simulink model "Foc_2024b"  (R2025a)
settings: Solver=FixedStepDiscrete  StartTime=0.0  StopTime=10.0  FixedStep=0.001  RelTol=1e-3
values from neighbouring files (symbols this model uses):
  cal_AdcMaxCountsHw = NoneSAR.Parameter    [Foc_2024b_LoadCalParameter.m]
  cal_AdcRefVoltHw = NoneSAR.Parameter    [Foc_2024b_LoadCalParameter.m]
  cal_AdcVoltMidHw = NoneSAR.Parameter    [Foc_2024b_LoadCalParameter.m]
  cal_bActHwMode = NoneSAR.Parameter    [Foc_2024b_LoadCalParameter.m]    (also in Foc_LoadCalParameter.m)
  cal_FullScaleCur = NoneSAR.Parameter    [Foc_2024b_LoadCalParameter.m]
  cal_GainAmpHw = NoneSAR.Parameter    [Foc_2024b_LoadCalParameter.m]
  cal_HwtDutyU = NoneSAR.Parameter    [Foc_2024b_LoadCalParameter.m]
  cal_HwtDutyV = NoneSAR.Parameter    [Foc_2024b_LoadCalParameter.m]
  cal_HwtDutyW = NoneSAR.Parameter    [Foc_2024b_LoadCalParameter.m]
  cal_HwtSector = NoneSAR.Parameter    [Foc_2024b_LoadCalParameter.m]
  cal_OhmRShuntHw = NoneSAR.Parameter    [Foc_2024b_LoadCalParameter.m]
  cal_s16Inductivity = NoneSAR.Parameter    [Foc_2024b_LoadCalParameter.m]    (also in Foc_LoadCalParameter.m)
  cal_s16LpfPllEst = NoneSAR.Parameter    [Foc_2024b_LoadCalParameter.m]    (also in Foc_LoadCalParameter.m)
  cal_s16LpfPllEstOpenLoop = NoneSAR.Parameter    [Foc_2024b_LoadCalParameter.m]    (also in Foc_LoadCalParameter.m)
  cal_s16MinSampleTime = NoneSAR.Parameter    [Foc_2024b_LoadCalParameter.m]    (also in Foc_LoadCalParameter.m)
  cal_s16OmegaGainEst = NoneSAR.Parameter    [Foc_2024b_LoadCalParameter.m]    (also in Foc_LoadCalParameter.m)
  cal_s16RPha = NoneSAR.Parameter    [Foc_2024b_LoadCalParameter.m]    (also in Foc_LoadCalParameter.m)
  cal_s16ThresholdPhaCurImplaisible = NoneSAR.Parameter    [Foc_2024b_LoadCalParameter.m]    (also in Foc_LoadCalParameter.m)
  cal_u8TiDebPhaCur = NoneSAR.Parameter    [Foc_2024b_LoadCalParameter.m]    (also in Foc_LoadCalParameter.m)
undefined symbols (not defined in the file or in its folder): AdcTriggerOffset, CCU6_T12PERIOD, CCU_PWM_PERIOD_TICKS_HALF, DCLINK_VOLTAGE_FACTOR, DesiredPwm_U, DesiredPwm_V, DesiredPwm_W, e_motorstate_t, e_running_dir_t, FOC_SVM_MAX, FOC_VD_VQ_MAX, FOC_VD_VQ_MAX_100, FOC_VD_VQ_MAX_95, FOC_VD_VQ_MAX_97, FOCLLD_CCU_PWM_PERIOD_TICKS_HALF, FOCLLD_SKIP_DEAD_TIME_THRESHOLD, MAX_DUTY, MIN_SAMPLE_TIME_DEFAULT, MODULATION_FLATBOTTOM, ONEBY_CURRENT_AMPLIFICATION, PhaseCurrentU, PhaseCurrentV, PhaseCurrentW, PwmShift_DutyLong, PwmShift_DutyMed, PwmShift_DutyShort, PwmShiftPtr_RiseLong, PwmShiftPtr_RiseMed, PwmShiftPtr_RiseShort, s16_EST_THETA_GAIN, s16_ONEBYSQR3, s16_SQR3OVER2, st_c_pi_Q_s16_outMax, st_c_pi_Q_s16_outMin, U8_INDUCTIVITY_FAC, VQ_MAX_TABLE_SIZE, VqMaxTable_100, VqMaxTable_95, VqMaxTable_97
libraries: simulink x16, hdlsllib x2
(part 1 of 6)
settings Model: Creator=sg179620  LastModifiedBy=wangtianqi
settings OptimizationCC: DefaultParameterBehavior=Inlined  EnhancedBackFolding=on  PassReuseOutputArgsAs=Individual arguments  ZeroExternalMemoryAtStartup=off  ZeroInternalMemoryAtStartup=off  OptimizeBlockOrder=speed  DifferentSizesBufferReuse=on  OptimizationCustomize=off  EfficientTunableParamExpr=on
settings DebuggingCC: ParameterTunabilityLossMsg=error
settings SFSimCC: MATLABDynamicMemAlloc=off
settings RTWCC: SystemTargetFile=ert.tlc  TemplateMakefile=ert_default_tmf  Description=Embedded Coder
settings CodeAppCC: ForceParamTrailComments=on  IgnoreCustomStorageClasses=off  OperatorAnnotations=on  SimulinkDataObjDesc=on  SFDataObjDesc=on  InsertBlockDesc=on
settings ERTTargetCC: ExtModeTransport=0.0  ExtModeStaticAlloc=off  ExtModeMexFile=ext_comm  ExtModeIntrfLevel=Level1  ERTCustomFileTemplate=example_file_process.tlc  TargetLangStandard=C99 (ISO)  GenerateSampleERTMain=on

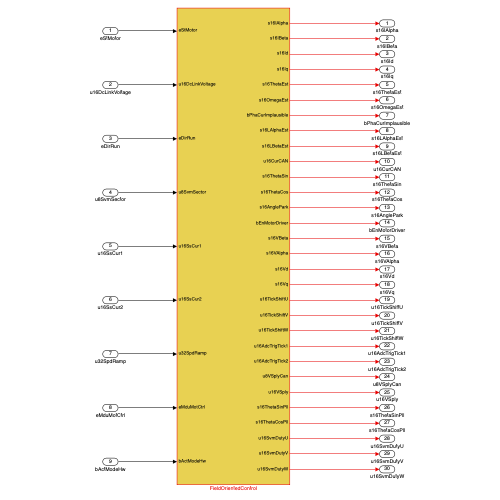
[thumbnail: Simulink's stored preview of the top-level diagram]
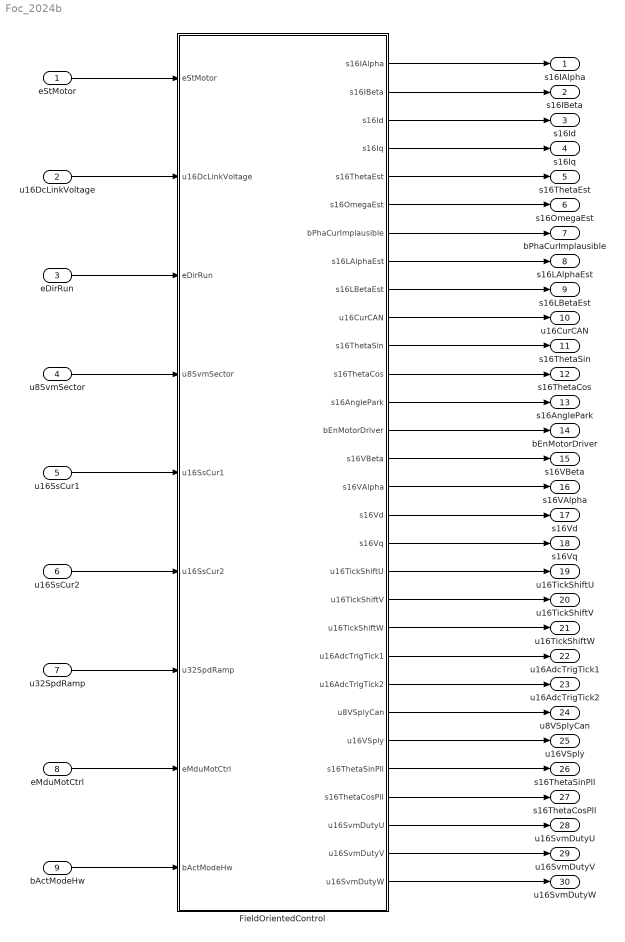
== system Foc_2024b ==
  eStMotor : Inport  OutDataTypeStr=Enum: auto
  u16DcLinkVoltage : Inport  Port=2  OutDataTypeStr=uint16
  eDirRun : Inport  Port=3  OutDataTypeStr=Enum: auto
  u8SvmSector : Inport  Port=4  OutDataTypeStr=uint8
  u16SsCur1 : Inport  Port=5  OutDataTypeStr=uint16
  u16SsCur2 : Inport  Port=6  OutDataTypeStr=uint16
  u32SpdRamp : Inport  Port=7  OutDataTypeStr=uint32
  eMduMotCtrl : Inport  Port=8  OutDataTypeStr=Enum: auto
  bActModeHw : Inport  Port=9  OutDataTypeStr=boolean
  FieldOrientedControl : Subsystem
  s16IAlpha : Outport  OutDataTypeStr=int16
  s16IBeta : Outport  Port=2  OutDataTypeStr=int16
  s16Id : Outport  Port=3  OutDataTypeStr=int16
  s16Iq : Outport  Port=4  OutDataTypeStr=int16
  s16ThetaEst : Outport  Port=5  OutDataTypeStr=int16
  s16OmegaEst : Outport  Port=6  OutDataTypeStr=int16
  bPhaCurImplausible : Outport  Port=7  OutDataTypeStr=boolean
  s16LAlphaEst : Outport  Port=8  OutDataTypeStr=int16
  s16LBetaEst : Outport  Port=9  OutDataTypeStr=int16
  u16CurCAN : Outport  Port=10  OutDataTypeStr=uint16
  s16ThetaSin : Outport  Port=11  OutDataTypeStr=int16
  s16ThetaCos : Outport  Port=12  OutDataTypeStr=int16
  s16AnglePark : Outport  Port=13  OutDataTypeStr=int16
  bEnMotorDriver : Outport  Port=14  OutDataTypeStr=boolean
  s16VBeta : Outport  Port=15  OutDataTypeStr=int16
  s16VAlpha : Outport  Port=16  OutDataTypeStr=int16
  s16Vd : Outport  Port=17  OutDataTypeStr=int16
  s16Vq : Outport  Port=18  OutDataTypeStr=int16
  u16TickShiftU : Outport  Port=19  OutDataTypeStr=uint16
  u16TickShiftV : Outport  Port=20  OutDataTypeStr=uint16
  u16TickShiftW : Outport  Port=21  OutDataTypeStr=uint16
  u16AdcTrigTick1 : Outport  Port=22  OutDataTypeStr=uint16
  u16AdcTrigTick2 : Outport  Port=23  OutDataTypeStr=uint16
  u8VSplyCan : Outport  Port=24  OutDataTypeStr=uint8
  u16VSply : Outport  Port=25  OutDataTypeStr=uint16
  s16ThetaSinPll : Outport  Port=26  OutDataTypeStr=int16
  s16ThetaCosPll : Outport  Port=27  OutDataTypeStr=int16
  u16SvmDutyU : Outport  Port=28  OutDataTypeStr=uint16
  u16SvmDutyV : Outport  Port=29  OutDataTypeStr=uint16
  u16SvmDutyW : Outport  Port=30  OutDataTypeStr=uint16
  wires:
  eStMotor/1 -> FieldOrientedControl/1(eStMotor)
  u16DcLinkVoltage/1 -> FieldOrientedControl/2(u16DcLinkVoltage)
  eDirRun/1 -> FieldOrientedControl/3(eDirRun)
  u8SvmSector/1 -> FieldOrientedControl/4(u8SvmSector)
  u16SsCur1/1 -> FieldOrientedControl/5(u16SsCur1)
  u16SsCur2/1 -> FieldOrientedControl/6(u16SsCur2)
  bActModeHw/1 -> FieldOrientedControl/9(bActModeHw)
  u32SpdRamp/1 -> FieldOrientedControl/7(u32SpdRamp)
  eMduMotCtrl/1 -> FieldOrientedControl/8(eMduMotCtrl)
  FieldOrientedControl/1(s16IAlpha) -> s16IAlpha/1
  FieldOrientedControl/8(s16LAlphaEst) -> s16LAlphaEst/1
  FieldOrientedControl/6(s16OmegaEst) -> s16OmegaEst/1
  FieldOrientedControl/4(s16Iq) -> s16Iq/1
  FieldOrientedControl/2(s16IBeta) -> s16IBeta/1
  FieldOrientedControl/9(s16LBetaEst) -> s16LBetaEst/1
  FieldOrientedControl/7(bPhaCurImplausible) -> bPhaCurImplausible/1
  FieldOrientedControl/5(s16ThetaEst) -> s16ThetaEst/1
  FieldOrientedControl/3(s16Id) -> s16Id/1
  FieldOrientedControl/16(s16VAlpha) -> s16VAlpha/1
  FieldOrientedControl/14(bEnMotorDriver) -> bEnMotorDriver/1
  FieldOrientedControl/12(s16ThetaCos) -> s16ThetaCos/1
  FieldOrientedControl/10(u16CurCAN) -> u16CurCAN/1
  FieldOrientedControl/17(s16Vd) -> s16Vd/1
  FieldOrientedControl/15(s16VBeta) -> s16VBeta/1
  FieldOrientedControl/13(s16AnglePark) -> s16AnglePark/1
  FieldOrientedControl/11(s16ThetaSin) -> s16ThetaSin/1
  FieldOrientedControl/24(u8VSplyCan) -> u8VSplyCan/1
  FieldOrientedControl/22(u16AdcTrigTick1) -> u16AdcTrigTick1/1
  FieldOrientedControl/20(u16TickShiftV) -> u16TickShiftV/1
  FieldOrientedControl/18(s16Vq) -> s16Vq/1
  FieldOrientedControl/25(u16VSply) -> u16VSply/1
  FieldOrientedControl/23(u16AdcTrigTick2) -> u16AdcTrigTick2/1
  FieldOrientedControl/21(u16TickShiftW) -> u16TickShiftW/1
  FieldOrientedControl/19(u16TickShiftU) -> u16TickShiftU/1
  FieldOrientedControl/30(u16SvmDutyW) -> u16SvmDutyW/1
  FieldOrientedControl/28(u16SvmDutyU) -> u16SvmDutyU/1
  FieldOrientedControl/26(s16ThetaSinPll) -> s16ThetaSinPll/1
  FieldOrientedControl/29(u16SvmDutyV) -> u16SvmDutyV/1
  FieldOrientedControl/27(s16ThetaCosPll) -> s16ThetaCosPll/1

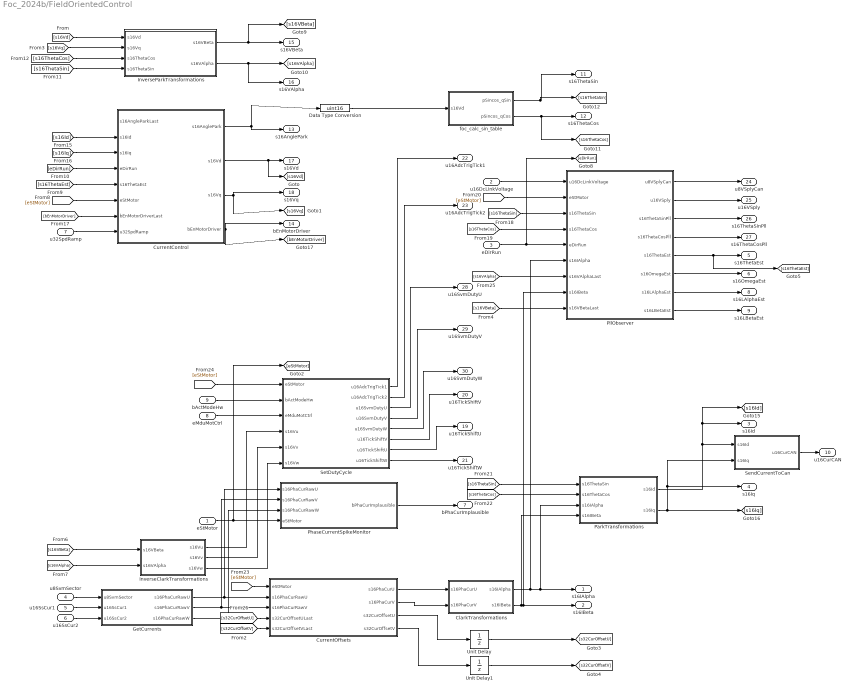
== system Foc_2024b/FieldOrientedControl ==
  eStMotor : Inport  OutDataTypeStr=Enum: auto
  u16DcLinkVoltage : Inport  Port=2  OutDataTypeStr=uint16
  eDirRun : Inport  Port=3  OutDataTypeStr=Enum: auto
  u8SvmSector : Inport  Port=4  OutDataTypeStr=uint8
  u16SsCur1 : Inport  Port=5  OutDataTypeStr=uint16
  u16SsCur2 : Inport  Port=6  OutDataTypeStr=uint16
  u32SpdRamp : Inport  Port=7  OutDataTypeStr=uint32
  eMduMotCtrl : Inport  Port=8  OutDataTypeStr=Enum: auto
  bActModeHw : Inport  Port=9  OutDataTypeStr=boolean
  ClarkTransformations : Subsystem
  CurrentControl : Subsystem
  CurrentOffsets : Subsystem  Description=Calculate current offsets.
  Data Type Conversion : DataTypeConversion  OutDataTypeStr=uint16  SaturateOnIntegerOverflow=off  RndMeth=Floor
  GetCurrents : Subsystem  Description=Reconstruct the 3 Phase Currents from single shunt measurement, basing upon svm sector.
  InverseClarkTransformations : Subsystem
  InverseParkTransformations : Subsystem
  ParkTransformations : Subsystem
  PhaseCurrentSpikeMonitor : Subsystem  Description=|  TreatAsAtomicUnit=on  RTWFcnName=phase_current_spike_monitor
      | This diagnosis is used to detect a faulty commutation due to high and short phase currents spike
      | This can also be  used to detect an implausible phase current.
      settings: RTWFcnNameOpts=User specified
  PllObserver : Subsystem  TreatAsAtomicUnit=on  RTWFcnName=motor_foc_pll_observer
      settings: RTWSystemCode=Nonreusable function  RTWFcnNameOpts=User specified
  SendCurrentToCan : Subsystem
  SetDutyCycle : Subsystem
  Unit Delay : UnitDelay  SampleTime=-1  HasFrameUpgradeWarning=on
  Unit Delay1 : UnitDelay  SampleTime=-1  HasFrameUpgradeWarning=on
  foc_calc_sin_table : Subsystem
  s16IAlpha : Outport  OutDataTypeStr=int16
  s16IBeta : Outport  Port=2  OutDataTypeStr=int16
  s16Id : Outport  Port=3  OutDataTypeStr=int16
  s16Iq : Outport  Port=4  OutDataTypeStr=int16
  s16ThetaEst : Outport  Port=5  OutDataTypeStr=int16
  s16OmegaEst : Outport  Port=6  OutDataTypeStr=int16
  bPhaCurImplausible : Outport  Port=7  OutDataTypeStr=boolean
  s16LAlphaEst : Outport  Port=8  OutDataTypeStr=int16
  s16LBetaEst : Outport  Port=9  OutDataTypeStr=int16
  u16CurCAN : Outport  Port=10  OutDataTypeStr=uint16
  s16ThetaSin : Outport  Port=11  OutDataTypeStr=int16
  s16ThetaCos : Outport  Port=12  OutDataTypeStr=int16
  s16AnglePark : Outport  Port=13  OutDataTypeStr=int16
  bEnMotorDriver : Outport  Port=14  OutDataTypeStr=boolean
  s16VBeta : Outport  Port=15  OutDataTypeStr=int16
  s16VAlpha : Outport  Port=16  OutDataTypeStr=int16
  s16Vd : Outport  Port=17  OutDataTypeStr=int16
  s16Vq : Outport  Port=18  OutDataTypeStr=int16
  u16TickShiftU : Outport  Port=19  OutDataTypeStr=uint16
  u16TickShiftV : Outport  Port=20  OutDataTypeStr=uint16
  u16TickShiftW : Outport  Port=21  OutDataTypeStr=uint16
  u16AdcTrigTick1 : Outport  Port=22  OutDataTypeStr=uint16
  u16AdcTrigTick2 : Outport  Port=23  OutDataTypeStr=uint16
  u8VSplyCan : Outport  Port=24  OutDataTypeStr=uint8
  u16VSply : Outport  Port=25  OutDataTypeStr=uint16
  s16ThetaSinPll : Outport  Port=26  OutDataTypeStr=int16
  s16ThetaCosPll : Outport  Port=27  OutDataTypeStr=int16
  u16SvmDutyU : Outport  Port=28  OutDataTypeStr=uint16
  u16SvmDutyV : Outport  Port=29  OutDataTypeStr=uint16
  u16SvmDutyW : Outport  Port=30  OutDataTypeStr=uint16
  wires:
  [eDirRun] -> CurrentControl/4(eDirRun)
  Unit Delay/1 -> [s32CurOffsetU]
  [s32CurOffsetV] -> CurrentOffsets/5(s32CurOffsetVLast)
  [s16Iq] -> CurrentControl/3(s16Iq)
  [s16ThetaCos] -> PllObserver/4(s16ThetaCos)
  [s16Vd] -> InverseParkTransformations/1(s16Vd)
  [s16Id] -> CurrentControl/2(s16Id)
  [bEnMotorDriver] -> CurrentControl/7(bEnMotorDriverLast)
  [s16ThetaSin] -> InverseParkTransformations/4(s16ThetaSin)
  [s16ThetaSin] -> PllObserver/3(s16ThetaSin)
  Data Type Conversion/1 -> foc_calc_sin_table/1(s16Vd)
  [s16ThetaCos] -> InverseParkTransformations/3(s16ThetaCos)
  [s16VBeta] -> PllObserver/9(s16VBetaLast)
  [eStMotor] -> PllObserver/2(eStMotor)
  [eStMotor] -> SetDutyCycle/1(eStMotor)
  [s16ThetaEst] -> CurrentControl/5(s16ThetaEst)
  [eStMotor] -> CurrentOffsets/1(eStMotor)
  GetCurrents/2(s16PhaCurRawV) -> CurrentOffsets/3(s16PhaCurRawV), PhaseCurrentSpikeMonitor/2(s16PhaCurRawV)
  [eStMotor] -> CurrentControl/6(eStMotor)
  [s16Vq] -> InverseParkTransformations/2(s16Vq)
  eMduMotCtrl/1 -> SetDutyCycle/3(eMduMotCtrl)
  bActModeHw/1 -> SetDutyCycle/2(bActModeHw)
  InverseParkTransformations/2(s16VAlpha) -> s16VAlpha/1, [s16VAlpha]
  u16SsCur2/1 -> GetCurrents/3(u16SsCur2)
  u32SpdRamp/1 -> CurrentControl/8(u32SpdRamp)
  [s16ThetaSin] -> ParkTransformations/1(s16ThetaSin)
  [s16VAlpha] -> PllObserver/7(s16VAlphaLast)
  foc_calc_sin_table/2(pSincos_qCos) -> [s16ThetaCos], s16ThetaCos/1
  foc_calc_sin_table/1(pSincos_qSin) -> [s16ThetaSin], s16ThetaSin/1
  [s16VBeta] -> InverseClarkTransformations/1(s16VBeta)
  [s16ThetaCos] -> ParkTransformations/2(s16ThetaCos)
  [s32CurOffsetU] -> CurrentOffsets/4(s32CurOffsetULast)
  SetDutyCycle/1(u16AdcTrigTick1) -> u16AdcTrigTick1/1
  [s16VAlpha] -> InverseClarkTransformations/2(s16VAlpha)
  eDirRun/1 -> [eDirRun], PllObserver/5(eDirRun)
  u16DcLinkVoltage/1 -> PllObserver/1(u16DcLinkVoltage)
  u16SsCur1/1 -> GetCurrents/2(u16SsCur1)
  u8SvmSector/1 -> GetCurrents/1(u8SvmSector)
  InverseParkTransformations/1(s16VBeta) -> s16VBeta/1, [s16VBeta]
  CurrentControl/1(s16AnglePark) -> Data Type Conversion/1, s16AnglePark/1
  CurrentControl/3(s16Vq) -> [s16Vq], s16Vq/1
  CurrentControl/2(s16Vd) -> s16Vd/1, [s16Vd]
  CurrentControl/4(bEnMotorDriver) -> bEnMotorDriver/1, [bEnMotorDriver]
  eStMotor/1 -> PhaseCurrentSpikeMonitor/4(eStMotor), [eStMotor]
  InverseClarkTransformations/1(s16Vu) -> SetDutyCycle/4(s16Vu)
  InverseClarkTransformations/2(s16Vv) -> SetDutyCycle/5(s16Vv)
  ClarkTransformations/2(s16IBeta) -> PllObserver/8(s16IBeta), s16IBeta/1, ParkTransformations/4(s16IBeta)
  InverseClarkTransformations/3(s16Vw) -> SetDutyCycle/6(s16Vw)
  GetCurrents/1(s16PhaCurRawU) -> CurrentOffsets/2(s16PhaCurRawU), PhaseCurrentSpikeMonitor/1(s16PhaCurRawU)
  ClarkTransformations/1(s16IAlpha) -> ParkTransformations/3(s16IAlpha), s16IAlpha/1, PllObserver/6(s16IAlpha)
  GetCurrents/3(s16PhaCurRawW) -> PhaseCurrentSpikeMonitor/3(s16PhaCurRawW)
  SetDutyCycle/2(u16AdcTrigTick2) -> u16AdcTrigTick2/1
  SetDutyCycle/3(u16SvmDutyU) -> u16SvmDutyU/1
  CurrentOffsets/1(s16PhaCurU) -> ClarkTransformations/1(s16PhaCurU)
  SetDutyCycle/4(u16SvmDutyV) -> u16SvmDutyV/1
  PhaseCurrentSpikeMonitor/1(bPhaCurImplausible) -> bPhaCurImplausible/1
  PllObserver/8(s16LBetaEst) -> s16LBetaEst/1
  SetDutyCycle/5(u16SvmDutyW) -> u16SvmDutyW/1
  SetDutyCycle/6(u16TickShiftV) -> u16TickShiftV/1
  PllObserver/7(s16LAlphaEst) -> s16LAlphaEst/1
  SetDutyCycle/7(u16TickShiftU) -> u16TickShiftU/1
  SetDutyCycle/8(u16TickShiftW) -> u16TickShiftW/1
  CurrentOffsets/2(s16PhaCurV) -> ClarkTransformations/2(s16PhaCurV)
  CurrentOffsets/3(s32CurOffsetU) -> Unit Delay/1
  Unit Delay1/1 -> [s32CurOffsetV]
  CurrentOffsets/4(s32CurOffsetV) -> Unit Delay1/1
  PllObserver/1(u8VSplyCan) -> u8VSplyCan/1
  PllObserver/2(u16VSply) -> u16VSply/1
  PllObserver/3(s16ThetaSinPll) -> s16ThetaSinPll/1
  PllObserver/4(s16ThetaCosPll) -> s16ThetaCosPll/1
  PllObserver/5(s16ThetaEst) -> [s16ThetaEst], s16ThetaEst/1
  PllObserver/6(s16OmegaEst) -> s16OmegaEst/1
  ParkTransformations/1(s16Id) -> s16Id/1, [s16Id], SendCurrentToCan/1(s16Id)
  ParkTransformations/2(s16Iq) -> s16Iq/1, SendCurrentToCan/2(s16Iq), [s16Iq]
  SendCurrentToCan/1(u16CurCAN) -> u16CurCAN/1

== system Foc_2024b/FieldOrientedControl/ClarkTransformations ==
  s16PhaCurU : Inport  OutDataTypeStr=int16
  s16PhaCurV : Inport  Port=2  OutDataTypeStr=int16
  Add4 : Sum  OutDataTypeStr=fixdt(1,16,15)
  Constant10 : Constant  Value=s16_ONEBYSQR3  OutDataTypeStr=int16
  Constant11 : Constant  Value=2  OutDataTypeStr=int8
  Constant9 : Constant  Value=s16_ONEBYSQR3  OutDataTypeStr=int16
  Product : Product  OutDataTypeStr=fixdt(1,16,15)
  Product1 : Product  OutDataTypeStr=fixdt(1,16,15)
  Product2 : Product  OutDataTypeStr=int16
  s16IAlpha : Outport  OutDataTypeStr=int16
  s16IBeta : Outport  Port=2  OutDataTypeStr=int16
  wires:
  s16PhaCurV/1 -> Product1/1
  s16PhaCurU/1 -> Product/1, s16IAlpha/1
  Constant10/1 -> Product1/2
  Constant9/1 -> Product/2
  Product1/1 -> Product2/1
  Product/1 -> Add4/1
  Product2/1 -> Add4/2
  Constant11/1 -> Product2/2
  Add4/1 -> s16IBeta/1

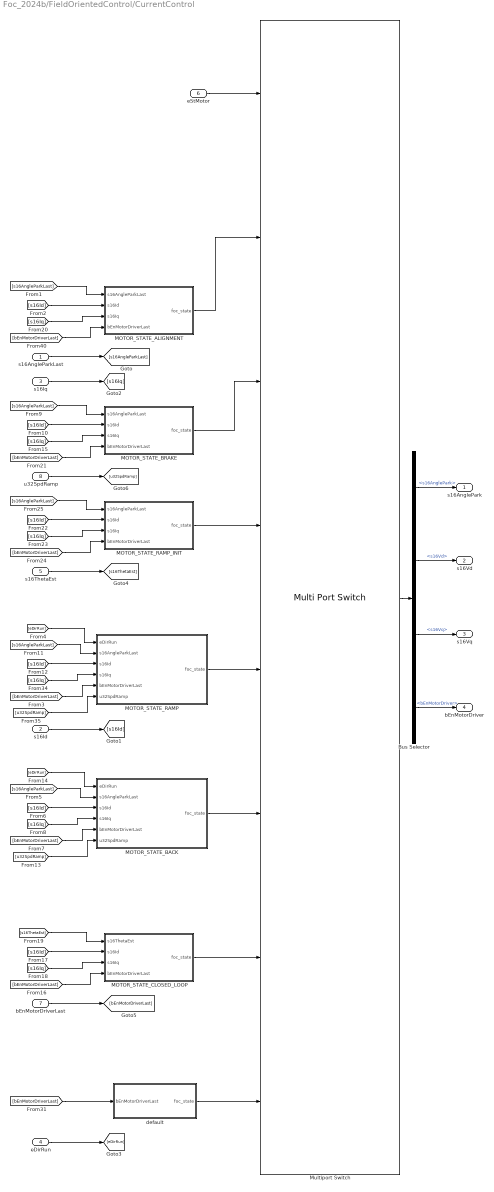
== system Foc_2024b/FieldOrientedControl/CurrentControl ==
  s16AngleParkLast : Inport  OutDataTypeStr=int16
  s16Id : Inport  Port=2  OutDataTypeStr=int16
  s16Iq : Inport  Port=3  OutDataTypeStr=int16
  eDirRun : Inport  Port=4  OutDataTypeStr=Enum: auto
  s16ThetaEst : Inport  Port=5  OutDataTypeStr=int16
  eStMotor : Inport  Port=6  OutDataTypeStr=Enum: auto
  bEnMotorDriverLast : Inport  Port=7  OutDataTypeStr=boolean
  u32SpdRamp : Inport  Port=8  OutDataTypeStr=uint32
  Bus Selector : BusSelector  OutputSignals=s16AnglePark,s16Vd,s16Vq,bEnMotorDriver
  MOTOR_STATE_ALIGNMENT : Subsystem
  MOTOR_STATE_BACK : Subsystem
  MOTOR_STATE_BRAKE : Subsystem
  MOTOR_STATE_CLOSED_LOOP : Subsystem
  MOTOR_STATE_RAMP : Subsystem
  MOTOR_STATE_RAMP_INIT : Subsystem
  Multiport Switch : MultiPortSwitch  DataPortOrder=Specify indices  DataPortIndices={e_motorstate_t.MOTOR_STATE_ALIGNMENT, e_motorstate_t.MOTOR_STATE_BRAKE, e_motorstate_t.MOTOR_STATE_RAMP_INIT, e_motorstate_t.MOTOR_STATE_RAMP, e_motorstate_t.MOTOR_STATE_BACK, e_motorstate_t.MOTOR_STATE_CLOSED_LOOP}  DataPortForDefault=Additional data port  DiagnosticForDefault=None  SaturateOnIntegerOverflow=off  InputSameDT=off
  default : Subsystem
  s16AnglePark : Outport  OutDataTypeStr=int16
  s16Vd : Outport  Port=2  OutDataTypeStr=int16
  s16Vq : Outport  Port=3  OutDataTypeStr=int16
  bEnMotorDriver : Outport  Port=4  OutDataTypeStr=boolean
  wires:
  [s16AngleParkLast] -> MOTOR_STATE_ALIGNMENT/1(s16AngleParkLast)
  [s16Id] -> MOTOR_STATE_ALIGNMENT/2(s16Id)
  [s16AngleParkLast] -> MOTOR_STATE_BRAKE/1(s16AngleParkLast)
  [s16Iq] -> MOTOR_STATE_ALIGNMENT/3(s16Iq)
  s16Iq/1 -> [s16Iq]
  [bEnMotorDriverLast] -> MOTOR_STATE_ALIGNMENT/4(bEnMotorDriverLast)
  s16AngleParkLast/1 -> [s16AngleParkLast]
  [s16Id] -> MOTOR_STATE_BRAKE/2(s16Id)
  [s16Iq] -> MOTOR_STATE_BRAKE/3(s16Iq)
  [bEnMotorDriverLast] -> MOTOR_STATE_BRAKE/4(bEnMotorDriverLast)
  u32SpdRamp/1 -> [u32SpdRamp]
  [s16AngleParkLast] -> MOTOR_STATE_RAMP_INIT/1(s16AngleParkLast)
  [s16Id] -> MOTOR_STATE_RAMP_INIT/2(s16Id)
  [s16Iq] -> MOTOR_STATE_RAMP_INIT/3(s16Iq)
  [bEnMotorDriverLast] -> MOTOR_STATE_RAMP_INIT/4(bEnMotorDriverLast)
  s16ThetaEst/1 -> [s16ThetaEst]
  [eDirRun] -> MOTOR_STATE_RAMP/1(eDirRun)
  [s16AngleParkLast] -> MOTOR_STATE_RAMP/2(s16AngleParkLast)
  [s16Id] -> MOTOR_STATE_RAMP/3(s16Id)
  [s16Iq] -> MOTOR_STATE_RAMP/4(s16Iq)
  [bEnMotorDriverLast] -> MOTOR_STATE_RAMP/5(bEnMotorDriverLast)
  [u32SpdRamp] -> MOTOR_STATE_RAMP/6(u32SpdRamp)
  s16Id/1 -> [s16Id]
  [eDirRun] -> MOTOR_STATE_BACK/1(eDirRun)
  [s16AngleParkLast] -> MOTOR_STATE_BACK/2(s16AngleParkLast)
  [s16Id] -> MOTOR_STATE_BACK/3(s16Id)
  [s16Iq] -> MOTOR_STATE_BACK/4(s16Iq)
  [bEnMotorDriverLast] -> MOTOR_STATE_BACK/5(bEnMotorDriverLast)
  MOTOR_STATE_RAMP/1(foc_state) -> Multiport Switch/5
  [u32SpdRamp] -> MOTOR_STATE_BACK/6(u32SpdRamp)
  [s16ThetaEst] -> MOTOR_STATE_CLOSED_LOOP/1(s16ThetaEst)
  [s16Id] -> MOTOR_STATE_CLOSED_LOOP/2(s16Id)
  [s16Iq] -> MOTOR_STATE_CLOSED_LOOP/3(s16Iq)
  [bEnMotorDriverLast] -> MOTOR_STATE_CLOSED_LOOP/4(bEnMotorDriverLast)
  bEnMotorDriverLast/1 -> [bEnMotorDriverLast]
  Multiport Switch/1 -> Bus Selector/1
  [bEnMotorDriverLast] -> default/1(bEnMotorDriverLast)
  eDirRun/1 -> [eDirRun]
  eStMotor/1 -> Multiport Switch/1
  MOTOR_STATE_BACK/1(foc_state) -> Multiport Switch/6
  MOTOR_STATE_ALIGNMENT/1(foc_state) -> Multiport Switch/2
  MOTOR_STATE_BRAKE/1(foc_state) -> Multiport Switch/3
  MOTOR_STATE_RAMP_INIT/1(foc_state) -> Multiport Switch/4
  MOTOR_STATE_CLOSED_LOOP/1(foc_state) -> Multiport Switch/7
  default/1(foc_state) -> Multiport Switch/8
  Bus Selector/1 -> s16AnglePark/1  "<s16AnglePark>"
  Bus Selector/3 -> s16Vq/1  "<s16Vq>"
  Bus Selector/2 -> s16Vd/1  "<s16Vd>"
  Bus Selector/4 -> bEnMotorDriver/1  "<bEnMotorDriver>"

== system Foc_2024b/FieldOrientedControl/CurrentOffsets ==
  eStMotor : Inport  OutDataTypeStr=Enum: auto
  s16PhaCurRawU : Inport  Port=2  OutDataTypeStr=int16
  s16PhaCurRawV : Inport  Port=3  OutDataTypeStr=int16
  s32CurOffsetULast : Inport  Port=4  OutDataTypeStr=int32
  s32CurOffsetVLast : Inport  Port=5  OutDataTypeStr=int32
  Bus Creator : BusCreator  Inputs=4
  Bus Creator1 : BusCreator  Inputs=4
  Bus Selector : BusSelector  OutputSignals=s16PhaCurU,s16PhaCurV,s32CurOffsetU,s32CurOffsetV
  Enumerated Constant5 : simulink/Sources/Enumerated Constant  OutDataTypeStr=Enum: e_motorstate_t  Value=e_motorstate_t.MOTOR_STATE_OFF  SampleTime=inf
  If : If  IfExpression=u1
  Merge : Merge
  OffsetDefault : Subsystem  TreatAsAtomicUnit=on
  OffsetDetection : Subsystem  TreatAsAtomicUnit=on
  Relational Operator : RelationalOperator  Operator=~=  OutDataTypeStr=boolean  RndMeth=Simplest  InputSameDT=off
  s16PhaCurU : Outport  OutDataTypeStr=int16
  s16PhaCurV : Outport  Port=2  OutDataTypeStr=int16
  s32CurOffsetU : Outport  Port=3  OutDataTypeStr=int32
  s32CurOffsetV : Outport  Port=4  OutDataTypeStr=int32
  wires:
  eStMotor/1 -> Relational Operator/1
  s16PhaCurRawV/1 -> OffsetDetection/2(s16PhaCurRawV)
  s16PhaCurRawU/1 -> OffsetDetection/1(s16PhaCurRawU)
  Relational Operator/1 -> If/1
  Bus Selector/2 -> s16PhaCurV/1  "<s16PhaCurV>"
  Merge/1 -> Bus Selector/1
  Enumerated Constant5/1 -> Relational Operator/2
  If/2 -> OffsetDefault/Action
  Bus Selector/1 -> s16PhaCurU/1  "<s16PhaCurU>"
  If/1 -> OffsetDetection/Action
  Bus Creator/1 -> Merge/1
  s32CurOffsetULast/1 -> OffsetDetection/3(s32CurOffsetULast)
  Bus Creator1/1 -> Merge/2
  s32CurOffsetVLast/1 -> OffsetDetection/4(s32CurOffsetVLast)
  OffsetDetection/1(s16PhaCurU) -> Bus Creator/1  "s16PhaCurU"
  OffsetDetection/2(s16PhaCurV) -> Bus Creator/2  "s16PhaCurV"
  OffsetDetection/3(s32CurOffsetU) -> Bus Creator/3  "s32CurOffsetU"
  OffsetDetection/4(s32CurOffsetV) -> Bus Creator/4  "s32CurOffsetV"
  OffsetDefault/1(s16PhaCurU) -> Bus Creator1/1  "s16PhaCurU"
  OffsetDefault/2(s16PhaCurV) -> Bus Creator1/2  "s16PhaCurV"
  OffsetDefault/3(s32CurOffsetU) -> Bus Creator1/3  "s32CurOffsetU"
  OffsetDefault/4(s32CurOffsetV) -> Bus Creator1/4  "s32CurOffsetV"
  Bus Selector/3 -> s32CurOffsetU/1  "<s32CurOffsetU>"
  Bus Selector/4 -> s32CurOffsetV/1  "<s32CurOffsetV>"

== system Foc_2024b/FieldOrientedControl/GetCurrents ==
  u8SvmSector : Inport  OutDataTypeStr=uint8
  u16SsCur1 : Inport  Port=2  OutDataTypeStr=uint16
  u16SsCur2 : Inport  Port=3  OutDataTypeStr=uint16
  AdcVolToCur : Subsystem  Description=Coverts the orignal ADC voltage to current.
  Bus Creator{,1..5} (6 alike) : BusCreator  Inputs=3
  Bus Creator6 : BusCreator  Inputs=PhaseCurrentU,PhaseCurrentV,PhaseCurrentW
  Bus Selector : BusSelector  OutputSignals=PhaseCurrentU,PhaseCurrentV,PhaseCurrentW
  DEFAULT : Subsystem  Description=Default reconstruction  TreatAsAtomicUnit=on
  Merge : Merge  Inputs=7
  SECTOR_1 : Subsystem  Description=Sector1 reconstruction  TreatAsAtomicUnit=on
  SECTOR_2 : Subsystem  Description=Sector2 reconstruction  TreatAsAtomicUnit=on
  SECTOR_3 : Subsystem  Description=Sector3 reconstruction  TreatAsAtomicUnit=on
  SECTOR_4 : Subsystem  Description=Sector4 reconstruction  TreatAsAtomicUnit=on
  SECTOR_5 : Subsystem  Description=Sector5 reconstruction  TreatAsAtomicUnit=on
  SECTOR_6 : Subsystem  Description=Sector6 reconstruction  TreatAsAtomicUnit=on
  Switch Case : SwitchCase  CaseConditions={1,2,3,4,5,6}
  s16PhaCurRawU : Outport  OutDataTypeStr=int16
  s16PhaCurRawV : Outport  Port=2  OutDataTypeStr=int16
  s16PhaCurRawW : Outport  Port=3  OutDataTypeStr=int16
  wires:
  [s16SsCur1] -> SECTOR_6/1(s16SsCur1)
  [s16SsCur1] -> SECTOR_5/1(s16SsCur1)
  [s16SsCur1] -> SECTOR_3/1(s16SsCur1)
  [s16SsCur2] -> SECTOR_3/2(s16SsCur2)
  [s16SsCur1] -> SECTOR_2/1(s16SsCur1)
  [s16SsCur2] -> SECTOR_2/2(s16SsCur2)
  [s16SsCur2] -> SECTOR_6/2(s16SsCur2)
  [s16SsCur2] -> SECTOR_4/2(s16SsCur2)
  [s16SsCur2] -> SECTOR_1/2(s16SsCur2)
  SECTOR_4/1(s16PhaCurU) -> Bus Creator3/1  "PhaCurU"
  AdcVolToCur/2(s16SsCur2) -> [s16SsCur2]
  [s16SsCur2] -> SECTOR_5/2(s16SsCur2)
  [s16SsCur1] -> SECTOR_4/1(s16SsCur1)
  [s16SsCur1] -> SECTOR_1/1(s16SsCur1)
  u16SsCur2/1 -> AdcVolToCur/2(u16SsCur2)
  u16SsCur1/1 -> AdcVolToCur/1(u16SsCur1)
  AdcVolToCur/1(s16SsCur1) -> [s16SsCur1]
  u8SvmSector/1 -> Switch Case/1
  Bus Creator1/1 -> Merge/2
  Switch Case/1 -> SECTOR_1/Action
  SECTOR_2/1(s16PhaCurU) -> Bus Creator1/1  "PhaCurU"
  Switch Case/2 -> SECTOR_2/Action
  Bus Creator4/1 -> Merge/5
  Switch Case/3 -> SECTOR_3/Action
  Switch Case/4 -> SECTOR_4/Action
  Switch Case/5 -> SECTOR_5/Action
  Switch Case/6 -> SECTOR_6/Action
  Bus Creator2/1 -> Merge/3
  Switch Case/7 -> DEFAULT/Action
  SECTOR_6/3(s16PhaCurW) -> Bus Creator5/3  "PhaCurW"
  SECTOR_1/1(s16PhaCurU) -> Bus Creator/1  "PhaCurU"
  SECTOR_5/2(s16PhaCurV) -> Bus Creator4/2  "PhaCurV"
  SECTOR_1/2(s16PhaCurV) -> Bus Creator/2  "PhaCurV"
  SECTOR_1/3(s16PhaCurW) -> Bus Creator/3  "PhaCurW"
  SECTOR_2/2(s16PhaCurV) -> Bus Creator1/2  "PhaCurV"
  SECTOR_2/3(s16PhaCurW) -> Bus Creator1/3  "PhaCurW"
  SECTOR_3/1(s16PhaCurU) -> Bus Creator2/1  "PhaCurU"
  SECTOR_3/2(s16PhaCurV) -> Bus Creator2/2  "PhaCurV"
  SECTOR_3/3(s16PhaCurW) -> Bus Creator2/3  "PhaCurW"
  SECTOR_4/2(s16PhaCurV) -> Bus Creator3/2  "PhaCurV"
  SECTOR_4/3(s16PhaCurW) -> Bus Creator3/3  "PhaCurW"
  DEFAULT/1(s16PhaCurU) -> Bus Creator6/1  "PhaCurU"
  Bus Creator6/1 -> Merge/7
  DEFAULT/2(s16PhaCurV) -> Bus Creator6/2  "PhaCurV"
  DEFAULT/3(s16PhaCurW) -> Bus Creator6/3  "PhaCurW"
  SECTOR_5/1(s16PhaCurU) -> Bus Creator4/1  "PhaCurU"
  SECTOR_5/3(s16PhaCurW) -> Bus Creator4/3  "PhaCurW"
  SECTOR_6/1(s16PhaCurU) -> Bus Creator5/1  "PhaCurU"
  SECTOR_6/2(s16PhaCurV) -> Bus Creator5/2  "PhaCurV"
  Bus Creator/1 -> Merge/1
  Bus Creator3/1 -> Merge/4
  Bus Selector/2 -> s16PhaCurRawV/1  "<PhaseCurrentV>"
  Bus Creator5/1 -> Merge/6
  Merge/1 -> Bus Selector/1
  Bus Selector/1 -> s16PhaCurRawU/1  "<PhaseCurrentU>"
  Bus Selector/3 -> s16PhaCurRawW/1  "<PhaseCurrentW>"

== system Foc_2024b/FieldOrientedControl/InverseClarkTransformations ==
  s16VBeta : Inport  OutDataTypeStr=int16
  s16VAlpha : Inport  Port=2  OutDataTypeStr=int16
  Add3 : Sum  Inputs=+-  OutDataTypeStr=fixdt(1,16,15)
  Add4 : Sum  Inputs=+-  OutDataTypeStr=fixdt(1,16,15)
  Constant3 : Constant  Value=s16_SQR3OVER2  OutDataTypeStr=fixdt(1,16,15)
  Constant4 : Constant  Value=2  OutDataTypeStr=int16
  Constant5 : Constant  Value=s16_SQR3OVER2  OutDataTypeStr=fixdt(1,16,15)
  Constant6 : Constant  Value=2  OutDataTypeStr=int16
  Constant7 : Constant  Value=-1  OutDataTypeStr=int16
  Divide : Product  Inputs=*/  OutDataTypeStr=fixdt(1,16,15)
  Divide1 : Product  Inputs=*/  OutDataTypeStr=fixdt(1,16,15)
  Product4 : Product  OutDataTypeStr=fixdt(1,16,15)
  Product5 : Product  OutDataTypeStr=fixdt(1,16,15)
  Product6 : Product  OutDataTypeStr=fixdt(1,16,15)
  s16Vu : Outport  OutDataTypeStr=int16
  s16Vv : Outport  Port=2  OutDataTypeStr=int16
  s16Vw : Outport  Port=3  OutDataTypeStr=int16
  wires:
  Constant6/1 -> Divide1/2
  Product5/1 -> Product6/2
  s16VAlpha/1 -> [s16VAlpha]
  [s16VBeta] -> Divide/1
  Divide1/1 -> Add4/2
  Constant3/1 -> Product4/2
  Constant5/1 -> Product5/2
  s16VBeta/1 -> [s16VBeta]
  [s16VAlpha] -> Product4/1
  Constant7/1 -> Product6/1
  [s16VAlpha] -> Product5/1
  Product4/1 -> Add3/1
  Constant4/1 -> Divide/2
  [s16VBeta] -> s16Vw/1
  Add3/1 -> s16Vv/1
  Product6/1 -> Add4/1
  [s16VBeta] -> Divide1/1
  Divide/1 -> Add3/2
  Add4/1 -> s16Vu/1

== system Foc_2024b/FieldOrientedControl/InverseParkTransformations ==
  s16Vd : Inport  OutDataTypeStr=int16
  s16Vq : Inport  Port=2  OutDataTypeStr=int16
  s16ThetaCos : Inport  Port=3  OutDataTypeStr=int16
  s16ThetaSin : Inport  Port=4  OutDataTypeStr=int16
  Add1 : Sum  Inputs=+-  OutDataTypeStr=fixdt(1,16,15)
  Add2 : Sum  Inputs=+-  OutDataTypeStr=fixdt(1,16,15)
  Product{,1..3} (4 alike) : Product  OutDataTypeStr=fixdt(1,16,15)
  s16VBeta : Outport  OutDataTypeStr=int16
  s16VAlpha : Outport  Port=2  OutDataTypeStr=int16
  wires:
  s16Vq/1 -> Product3/2, Product1/2
  [SincosFOC_qSin] -> Product1/1
  s16Vd/1 -> Product2/2, Product/2
  [SincosFOC_qCos] -> Product/1
  s16ThetaSin/1 -> [SincosFOC_qSin]
  [SincosFOC_qCos] -> Product3/1
  s16ThetaCos/1 -> [SincosFOC_qCos]
  [SincosFOC_qSin] -> Product2/1
  Product2/1 -> Add2/1
  Product3/1 -> Add2/2
  Add2/1 -> s16VBeta/1
  Product/1 -> Add1/1
  Product1/1 -> Add1/2
  Add1/1 -> s16VAlpha/1

== system Foc_2024b/FieldOrientedControl/ParkTransformations ==
  s16ThetaSin : Inport  OutDataTypeStr=int16
  s16ThetaCos : Inport  Port=2  OutDataTypeStr=int16
  s16IAlpha : Inport  Port=3  OutDataTypeStr=int16
  s16IBeta : Inport  Port=4  OutDataTypeStr=int16
  Add5 : Sum
  Add6 : Sum  Inputs=+-
  Product{3..6} (4 alike) : Product  OutDataTypeStr=fixdt(1,16,15)
  s16IAlpha1 : InportShadow  Port=3  OutDataTypeStr=int16
  s16IBeta1 : InportShadow  Port=4  OutDataTypeStr=int16
  s16Id : Outport  OutDataTypeStr=int16
  s16Iq : Outport  Port=2  OutDataTypeStr=int16
  wires:
  s16IBeta/1 -> Product3/1
  Product4/1 -> Add5/2
  s16ThetaCos/1 -> Product5/1, Product4/2
  Product3/1 -> Add5/1
  s16ThetaSin/1 -> Product6/1, Product3/2
  s16IAlpha/1 -> Product4/1
  s16IAlpha1/1 -> Product6/2
  s16IBeta1/1 -> Product5/2
  Product5/1 -> Add6/1
  Product6/1 -> Add6/2
  Add5/1 -> s16Id/1
  Add6/1 -> s16Iq/1

== system Foc_2024b/FieldOrientedControl/PhaseCurrentSpikeMonitor ==
  s16PhaCurRawU : Inport  OutDataTypeStr=int16
  s16PhaCurRawV : Inport  Port=2  OutDataTypeStr=int16
  s16PhaCurRawW : Inport  Port=3  OutDataTypeStr=int16
  eStMotor : Inport  Port=4  OutDataTypeStr=Enum: auto
  Constant : Constant  Value=0  OutDataTypeStr=int8
  Constant1 : Constant  Value=-1  OutDataTypeStr=int8
  Constant12 : Constant  Value=cal_u8TiDebPhaCur  OutDataTypeStr=uint8
  Constant2 : Constant  Value=0  OutDataTypeStr=int8
  Constant3 : Constant  Value=-1  OutDataTypeStr=int8
  Constant4 : Constant  Value=0  OutDataTypeStr=int8
  Constant5 : Constant  Value=-1  OutDataTypeStr=int8
  Constant6 : Constant  Value=false  OutDataTypeStr=boolean
  Constant7 : Constant  Value=cal_s16ThresholdPhaCurImplaisible
  Constant8 : Constant  Value=true  OutDataTypeStr=boolean
  Constant9 : Constant  Value=false  OutDataTypeStr=boolean
  Enumerated Constant : simulink/Sources/Enumerated Constant  OutDataTypeStr=Enum: e_motorstate_t  Value=e_motorstate_t.MOTOR_STATE_OFF  SampleTime=inf
  Enumerated Constant1 : simulink/Sources/Enumerated Constant  OutDataTypeStr=Enum: e_motorstate_t  Value=e_motorstate_t.MOTOR_STATE_FINAL_OFF  SampleTime=inf
  Logical Operator : Logic  AllPortsSameDT=off  OutDataTypeStr=boolean
  Max : MinMax  Function=max  Inputs=3
  Product : Product  OutDataTypeStr=int16
  Product1 : Product  OutDataTypeStr=int16
  Product2 : Product  OutDataTypeStr=int16
  Relational Operator : RelationalOperator  Operator=<  OutDataTypeStr=boolean  RndMeth=Simplest  InputSameDT=off
  Relational Operator1 : RelationalOperator  Operator=<  OutDataTypeStr=boolean  RndMeth=Simplest  InputSameDT=off
  Relational Operator2 : RelationalOperator  Operator=<  OutDataTypeStr=boolean  RndMeth=Simplest  InputSameDT=off
  Relational Operator3 : RelationalOperator  Operator=~=  OutDataTypeStr=boolean  RndMeth=Simplest  InputSameDT=off
  Relational Operator4 : RelationalOperator  Operator=~=  OutDataTypeStr=boolean  RndMeth=Simplest  InputSameDT=off
  Relational Operator5 : RelationalOperator  Operator=>  OutDataTypeStr=boolean  RndMeth=Simplest  InputSameDT=off
  Switch{,1..4} (5 alike) : Switch  Criteria=u2 ~= 0  SaturateOnIntegerOverflow=off  InputSameDT=off
  "b_fault_debounce " : Subsystem
  bPhaCurImplausible : Outport  OutDataTypeStr=boolean
  wires:
  Constant5/1 -> Product2/1
  s16PhaCurRawW/1 -> Switch2/3, Relational Operator2/1, Product2/2
  Constant2/1 -> Relational Operator1/2
  Constant4/1 -> Relational Operator2/2
  s16PhaCurRawV/1 -> Switch1/3, Product1/2, Relational Operator1/1
  s16PhaCurRawU/1 -> Switch/3, Product/2, Relational Operator/1
  Constant3/1 -> Product1/1
  Constant7/1 -> Relational Operator5/2
  Constant/1 -> Relational Operator/2
  Constant8/1 -> Switch4/1
  Constant1/1 -> Product/1
  Relational Operator5/1 -> Switch4/2
  Relational Operator1/1 -> Switch1/2
  Product/1 -> Switch/1
  Relational Operator4/1 -> Logical Operator/2
  Relational Operator/1 -> Switch/2
  Relational Operator2/1 -> Switch2/2
  Product1/1 -> Switch1/1
  Relational Operator3/1 -> Logical Operator/1
  Product2/1 -> Switch2/1
  Switch/1 -> Max/1
  Max/1 -> Relational Operator5/1
  Switch1/1 -> Max/2
  Switch2/1 -> Max/3
  Enumerated Constant/1 -> Relational Operator3/1
  Constant6/1 -> Switch3/3
  eStMotor/1 -> Relational Operator4/1, Relational Operator3/2
  Enumerated Constant1/1 -> Relational Operator4/2
  Constant9/1 -> Switch4/3
  Switch4/1 -> Switch3/1
  Logical Operator/1 -> Switch3/2
  Switch3/1 -> "b_fault_debounce "/1(bSymptom)
  Constant12/1 -> "b_fault_debounce "/2(u8TiDeb)
  "b_fault_debounce "/1(bFlgFlt) -> bPhaCurImplausible/1

== system Foc_2024b/FieldOrientedControl/PllObserver ==
  u16DcLinkVoltage : Inport  OutDataTypeStr=uint16
  eStMotor : Inport  Port=2  OutDataTypeStr=Enum: auto
  s16ThetaSin : Inport  Port=3  OutDataTypeStr=int16
  s16ThetaCos : Inport  Port=4  OutDataTypeStr=int16
  eDirRun : Inport  Port=5  OutDataTypeStr=Enum: auto
  s16IAlpha : Inport  Port=6  OutDataTypeStr=int16
  s16VAlphaLast : Inport  Port=7  OutDataTypeStr=int16
  s16IBeta : Inport  Port=8  OutDataTypeStr=int16
  s16VBetaLast : Inport  Port=9  OutDataTypeStr=int16
  BackEMF : Subsystem  Description=Back EMF calculation for e_alpha and e_beta
  LowPassFilter : Subsystem
  ParkTransformationBEMF : Subsystem
  SinCosCalculation : Subsystem
  SupplyVoltageAdaptive : Subsystem
  ThetaOmegaCalculation : Subsystem  Description=|
      | theta, omega calculation
      | omega = (1/Kt)* (Eq - sgn(Eq)*Ed) (clockwise)
      | omega = (1/Kt)* (Eq + sgn(Eq)*Ed) (counterclockwise)
      | theta = theta + delta_theta
  Unit Delay : UnitDelay  SampleTime=-1  HasFrameUpgradeWarning=on
  u8VSplyCan : Outport  OutDataTypeStr=uint8
  u16VSply : Outport  Port=2  OutDataTypeStr=uint16
  s16ThetaSinPll : Outport  Port=3  OutDataTypeStr=int16
  s16ThetaCosPll : Outport  Port=4  OutDataTypeStr=int16
  s16ThetaEst : Outport  Port=5  OutDataTypeStr=int16
  s16OmegaEst : Outport  Port=6  OutDataTypeStr=int16
  s16LAlphaEst : Outport  Port=7  OutDataTypeStr=int16
  s16LBetaEst : Outport  Port=8  OutDataTypeStr=int16
  wires:
  s16IBeta/1 -> BackEMF/4(s16IBeta)
  s16VAlphaLast/1 -> BackEMF/3(s16VAlphaLast)
  BackEMF/4(s16EBetaEst) -> ParkTransformationBEMF/2(s16EBetaEst)
  s16IAlpha/1 -> BackEMF/2(s16IAlpha)
  s16VBetaLast/1 -> BackEMF/5(s16VBetaLast)
  u16DcLinkVoltage/1 -> SupplyVoltageAdaptive/1(u16DcLinkVoltage)
  SupplyVoltageAdaptive/3(u16VSply) -> u16VSply/1
  ParkTransformationBEMF/2(s16EqEst) -> LowPassFilter/2(s16EqEst)
  [s16ThetaEst] -> Unit Delay/1
  BackEMF/1(s16LAlphaEst) -> s16LAlphaEst/1
  SupplyVoltageAdaptive/1(s16VGainEst) -> BackEMF/1(s16VGainEst)
  SupplyVoltageAdaptive/2(u8VSplyCan) -> u8VSplyCan/1
  eStMotor/1 -> SinCosCalculation/1(eStMotor), [e_motorstate]
  Unit Delay/1 -> SinCosCalculation/2(s16ThetaEst)
  s16ThetaSin/1 -> SinCosCalculation/3(s16ThetaSin)
  LowPassFilter/1(s16EqFilterEst) -> ThetaOmegaCalculation/1(s16EqFilterEst)
  s16ThetaCos/1 -> SinCosCalculation/4(s16ThetaCos)
  eDirRun/1 -> ThetaOmegaCalculation/3(eDirRun)
  BackEMF/2(s16LBetaEst) -> s16LBetaEst/1
  BackEMF/3(s16EAlphaEst) -> ParkTransformationBEMF/1(s16EAlphaEst)
  SinCosCalculation/1(s16ThetaSinPll) -> ParkTransformationBEMF/3(s16ThetaSinPll), s16ThetaSinPll/1
  SinCosCalculation/2(s16ThetaCosPll) -> s16ThetaCosPll/1, ParkTransformationBEMF/4(s16ThetaCosPll)
  ParkTransformationBEMF/1(s16EdEst) -> LowPassFilter/1(s16EdEst)
  [e_motorstate] -> LowPassFilter/3(eStMotor)
  LowPassFilter/2(s16EdFilterEst) -> ThetaOmegaCalculation/2(s16EdFilterEst)
  ThetaOmegaCalculation/1(s16ThetaEst) -> [s16ThetaEst], s16ThetaEst/1
  ThetaOmegaCalculation/2(s16OmegaEst) -> s16OmegaEst/1

== system Foc_2024b/FieldOrientedControl/SendCurrentToCan ==
  s16Id : Inport  OutDataTypeStr=int16
  s16Iq : Inport  Port=2  OutDataTypeStr=int16
  Add : Sum
  Constant : Constant  Value=100  OutDataTypeStr=single
  Constant1 : Constant  Value=1.2247  OutDataTypeStr=single
  Data Type Conversion : DataTypeConversion  OutDataTypeStr=uint16  SaturateOnIntegerOverflow=off  RndMeth=Floor
  Divide{,1..3} (4 alike) : Product  Inputs=**
  Sqrt : Sqrt
  Subsystem : Subsystem
  Subsystem1 : Subsystem
  u16CurCAN : Outport  OutDataTypeStr=uint16
  wires:
  Constant/1 -> Divide2/2
  Sqrt/1 -> Divide3/1
  s16Id/1 -> Subsystem/1(In)
  Add/1 -> Divide2/1
  s16Iq/1 -> Subsystem1/1(In)
  Subsystem1/1(Out) -> Divide1/2, Divide1/1
  Subsystem/1(Out) -> Divide/2, Divide/1
  Divide1/1 -> Add/2
  Divide/1 -> Add/1
  Divide2/1 -> Sqrt/1
  Constant1/1 -> Divide3/2
  Divide3/1 -> Data Type Conversion/1
  Data Type Conversion/1 -> u16CurCAN/1

== system Foc_2024b/FieldOrientedControl/SetDutyCycle ==
  eStMotor : Inport  OutDataTypeStr=Enum: auto
  bActModeHw : Inport  Port=2  OutDataTypeStr=boolean
  eMduMotCtrl : Inport  Port=3  OutDataTypeStr=Enum: auto
  s16Vu : Inport  Port=4  OutDataTypeStr=int16
  s16Vv : Inport  Port=5  OutDataTypeStr=int16
  s16Vw : Inport  Port=6  OutDataTypeStr=int16
  PreCondition : Subsystem
  SetDuty : Subsystem
  u16AdcTrigTick1 : Outport  OutDataTypeStr=uint16
  u16AdcTrigTick2 : Outport  Port=2  OutDataTypeStr=uint16
  u16SvmDutyU : Outport  Port=3  OutDataTypeStr=uint16
  u16SvmDutyV : Outport  Port=4  OutDataTypeStr=uint16
  u16SvmDutyW : Outport  Port=5  OutDataTypeStr=uint16
  u16TickShiftV : Outport  Port=6  OutDataTypeStr=uint16
  u16TickShiftU : Outport  Port=7  OutDataTypeStr=uint16
  u16TickShiftW : Outport  Port=8  OutDataTypeStr=uint16
  wires:
  s16Vv/1 -> PreCondition/5(s16Vv)
  SetDuty/4(u16TickShiftU) -> u16TickShiftU/1
  eMduMotCtrl/1 -> PreCondition/3(eMduMotCtrl)
  eStMotor/1 -> PreCondition/1(eStMotor)
  PreCondition/1(stSvmDutyU) -> u16SvmDutyU/1, SetDuty/1(stSvmDutyU)
  s16Vw/1 -> PreCondition/6(s16Vw)
  s16Vu/1 -> PreCondition/4(s16Vu)
  bActModeHw/1 -> PreCondition/2(bActModeHw)
  PreCondition/2(u8SvmSector) -> SetDuty/2(u8SvmSector)
  PreCondition/3(stSvmDutyV) -> u16SvmDutyV/1, SetDuty/3(stSvmDutyV)
  SetDuty/2(u16AdcTrigTick2) -> u16AdcTrigTick2/1
  PreCondition/4(stSvmDutyW) -> SetDuty/4(stSvmDutyW), u16SvmDutyW/1
  SetDuty/1(u16AdcTrigTick1) -> u16AdcTrigTick1/1
  SetDuty/3(u16TickShiftV) -> u16TickShiftV/1
  SetDuty/5(u16TickShiftW) -> u16TickShiftW/1

== system Foc_2024b/FieldOrientedControl/foc_calc_sin_table ==
  s16Vd : Inport  OutDataTypeStr=int16
  Add : Sum  OutDataTypeStr=uint16
  Add1 : Sum  OutDataTypeStr=fixdt(1,16,15)
  Add2 : Sum  Inputs=+-
  Add3 : Sum
  Add4 : Sum  Inputs=+-
  Add5 : Sum  OutDataTypeStr=fixdt(1,16,15)
  Add6 : Sum  Inputs=+-  OutDataTypeStr=int16
  Add7 : Sum  OutDataTypeStr=int16
  Add8 : Sum  Inputs=+-
  Constant : Constant  Value=2^9  OutDataTypeStr=int16
  Constant1 : Constant  Value=2^9  OutDataTypeStr=int16
  Constant{2,4..5,7} (4 alike) : Constant  Value=512  OutDataTypeStr=int16
  Constant3 : Constant  OutDataTypeStr=uint8
  Constant6 : Constant  OutDataTypeStr=uint8
  Divide : Product  Inputs=*/  OutDataTypeStr=uint8
  Divide1 : Product  Inputs=*/  OutDataTypeStr=uint8
  Divide2 : Product  Inputs=*/
  Divide3 : Product  Inputs=*/
  Product : Product  OutDataTypeStr=uint16
  Product1 : Product  OutDataTypeStr=int16
  Product2 : Product  OutDataTypeStr=int16
  Product3 : Product  OutDataTypeStr=int16
  S16_SINUSTABLE : Lookup_n-D  NumberOfTableDimensions=1  BreakpointsForDimension1=[0:5]  IndexSearchMethod=Evenly spaced points  Table=[0:5]  ExtrapMethod=Clip  InputSameDT=off
  S16_SINUSTABLE1 : Lookup_n-D  NumberOfTableDimensions=1  BreakpointsForDimension1=[0:5]  Table=[0:5]  ExtrapMethod=Clip  InternalRulePriority=Speed  OutDataTypeStr=int16  RndMeth=Simplest  InputSameDT=off
  S16_SINUSTABLE2 : Lookup_n-D  NumberOfTableDimensions=1  BreakpointsForDimension1=[0:5]  Table=[0:5]  ExtrapMethod=Clip  InternalRulePriority=Speed  RndMeth=Simplest
  S16_SINUSTABLE3 : Lookup_n-D  NumberOfTableDimensions=1  BreakpointsForDimension1=[0:5]  Table=[0:5]  ExtrapMethod=Clip  InternalRulePriority=Speed  OutDataTypeStr=int16  RndMeth=Simplest  InputSameDT=off
  S16_SINUSTABLE4 : Lookup_n-D  NumberOfTableDimensions=1  BreakpointsForDimension1=[0:5]  Table=[0:5]  ExtrapMethod=Clip  InternalRulePriority=Speed  RndMeth=Simplest
  S16_SINUSTABLE5 : Lookup_n-D  NumberOfTableDimensions=1  BreakpointsForDimension1=[0:5]  Table=[0:5]  ExtrapMethod=Clip  InternalRulePriority=Speed  OutDataTypeStr=int16  RndMeth=Simplest  InputSameDT=off
  deg : Constant  Value=16384  OutDataTypeStr=int16
  pSincos_qSin : Outport
  pSincos_qCos : Outport  Port=2
  wires:
  S16_SINUSTABLE3/1 -> Add5/1
  s16Vd/1 -> Divide/1, [u16_sin_angle_sin], Add/1
  [u8_sin_sinpointer] -> Add3/1
  Constant3/1 -> Add3/2
  [u16_sin_angle_cos] -> Divide1/1
  Constant1/1 -> Divide1/2
  deg/1 -> Add/2
  [u8_sin_cospointer] -> Add7/1
  Constant6/1 -> Add7/2
  Constant/1 -> Divide/2
  Add3/1 -> S16_SINUSTABLE1/1
  Divide1/1 -> [u8_sin_cospointer]
  [u8_sin_sinpointer] -> S16_SINUSTABLE2/1
  S16_SINUSTABLE4/1 -> Add8/1
  Add/1 -> [u16_sin_angle_cos]
  Add7/1 -> S16_SINUSTABLE4/1
  [u8_sin_cospointer] -> S16_SINUSTABLE5/1
  Divide/1 -> [u8_sin_sinpointer]
  [u8_sin_sinpointer] -> Product/1
  Constant2/1 -> Product/2
  S16_SINUSTABLE1/1 -> Add4/1
  S16_SINUSTABLE2/1 -> Add4/2
  [u8_sin_cospointer] -> Product2/1
  Constant5/1 -> Product2/2
  S16_SINUSTABLE5/1 -> Add8/2
  [u16_sin_angle_sin] -> Add2/1
  Product/1 -> Add2/2
  Add4/1 -> Divide2/1
  Constant4/1 -> Divide2/2
  [u16_sin_angle_cos] -> Add6/1
  Product2/1 -> Add6/2
  Add8/1 -> Divide3/1
  Constant7/1 -> Divide3/2
  [u8_sin_sinpointer] -> S16_SINUSTABLE/1
  Add2/1 -> Product1/1
  Divide2/1 -> Product1/2
  [u8_sin_cospointer] -> S16_SINUSTABLE3/1
  Add6/1 -> Product3/1
  Divide3/1 -> Product3/2
  S16_SINUSTABLE/1 -> Add1/1
  Product1/1 -> Add1/2
  Product3/1 -> Add5/2
  Add1/1 -> pSincos_qSin/1
  Add5/1 -> pSincos_qCos/1

== system Foc_2024b/FieldOrientedControl/CurrentControl/MOTOR_STATE_ALIGNMENT ==
  s16AngleParkLast : Inport  OutDataTypeStr=int16
  s16Id : Inport  Port=2  OutDataTypeStr=int16
  s16Iq : Inport  Port=3  OutDataTypeStr=int16
  bEnMotorDriverLast : Inport  Port=4  OutDataTypeStr=boolean
  Compare To Constant : simulink/Logic and Bit Operations/Compare To Constant  relop===  const=false  OutDataTypeStr=boolean
  EnableDriver : Subsystem
  SetPiController : Subsystem
  Switch : Switch  Criteria=u2 ~= 0  SaturateOnIntegerOverflow=off  InputSameDT=off
  foc_state : Outport
  wires:
  bEnMotorDriverLast/1 -> [bEnMotorDriverLast]
  [bEnMotorDriverLast] -> Compare To Constant/1
  s16AngleParkLast/1 -> EnableDriver/1(s16AngleParkLast)
  s16Id/1 -> SetPiController/1(s16Id)
  s16Iq/1 -> SetPiController/2(s16Iq)
  [bEnMotorDriverLast] -> SetPiController/3(bEnMotorDriverLast)
  EnableDriver/1(foc_state) -> Switch/1
  Compare To Constant/1 -> Switch/2
  SetPiController/1(foc_state) -> Switch/3
  Switch/1 -> foc_state/1

== system Foc_2024b/FieldOrientedControl/CurrentControl/MOTOR_STATE_BACK ==
  eDirRun : Inport  OutDataTypeStr=Enum: auto
  s16AngleParkLast : Inport  Port=2  OutDataTypeStr=int16
  s16Id : Inport  Port=3  OutDataTypeStr=int16
  s16Iq : Inport  Port=4  OutDataTypeStr=int16
  bEnMotorDriverLast : Inport  Port=5  OutDataTypeStr=boolean
  u32SpdRamp : Inport  Port=6  OutDataTypeStr=uint32
  Bus Creator : BusCreator  Inputs=4
  PiCtrl_Calc_D : Subsystem
  "PiCtrl_Calc_Q " : Subsystem
  parkangle_cal : Subsystem
  foc_state : Outport
  wires:
  u32SpdRamp/1 -> parkangle_cal/2(u32SpdRamp)
  eDirRun/1 -> parkangle_cal/1(eDirRun)
  s16AngleParkLast/1 -> parkangle_cal/3(s16AngleParkLast)
  "PiCtrl_Calc_Q "/1(s16Vq) -> Bus Creator/3  "s16Vq"
  s16Id/1 -> PiCtrl_Calc_D/1(s16Id)
  s16Iq/1 -> "PiCtrl_Calc_Q "/1(s16Iq)
  parkangle_cal/1(s16AnglePark) -> Bus Creator/1  "s16AnglePark"
  PiCtrl_Calc_D/1(s16Vd) -> Bus Creator/2  "s16Vd"
  bEnMotorDriverLast/1 -> Bus Creator/4  "bEnMotorDriver"
  Bus Creator/1 -> foc_state/1

== system Foc_2024b/FieldOrientedControl/CurrentControl/MOTOR_STATE_BRAKE ==
  s16AngleParkLast : Inport  OutDataTypeStr=int16
  s16Id : Inport  Port=2  OutDataTypeStr=int16
  s16Iq : Inport  Port=3  OutDataTypeStr=int16
  bEnMotorDriverLast : Inport  Port=4  OutDataTypeStr=boolean
  Compare To Constant : simulink/Logic and Bit Operations/Compare To Constant  relop===  const=false  OutDataTypeStr=boolean
  EnableDriver : Subsystem
  SetPiController : Subsystem
  Switch : Switch  Criteria=u2 ~= 0  SaturateOnIntegerOverflow=off  InputSameDT=off
  foc_state : Outport
  wires:
  bEnMotorDriverLast/1 -> [bEnMotorDriverLast]
  s16AngleParkLast/1 -> EnableDriver/1(s16AngleParkLast)
  [bEnMotorDriverLast] -> Compare To Constant/1
  s16Id/1 -> SetPiController/1(s16Id)
  [bEnMotorDriverLast] -> SetPiController/3(bEnMotorDriverLast)
  s16Iq/1 -> SetPiController/2(s16Iq)
  EnableDriver/1(foc_state) -> Switch/1
  Compare To Constant/1 -> Switch/2
  SetPiController/1(foc_state) -> Switch/3
  Switch/1 -> foc_state/1

== system Foc_2024b/FieldOrientedControl/CurrentControl/MOTOR_STATE_CLOSED_LOOP ==
  s16ThetaEst : Inport  OutDataTypeStr=int16
  s16Id : Inport  Port=2  OutDataTypeStr=int16
  s16Iq : Inport  Port=3  OutDataTypeStr=int16
  bEnMotorDriverLast : Inport  Port=4  OutDataTypeStr=boolean
  " PiCtrl_Calc" : Subsystem
  Bus Creator : BusCreator  Inputs=4
  PIControl_update : Subsystem
  foc_state : Outport
  wires:
  Bus Creator/1 -> foc_state/1
  s16Id/1 -> " PiCtrl_Calc"/1(s16Id)
  s16Iq/1 -> PIControl_update/1(s16Iq)
  PIControl_update/1(s16Vq) -> Bus Creator/3  "s16Vq"
  s16ThetaEst/1 -> Bus Creator/1  "s16_foc_parkangle"
  " PiCtrl_Calc"/1(s16Vd) -> Bus Creator/2  "s16Vd"
  bEnMotorDriverLast/1 -> Bus Creator/4  "bEnMotorDriver"

== system Foc_2024b/FieldOrientedControl/CurrentControl/MOTOR_STATE_RAMP ==
  eDirRun : Inport  OutDataTypeStr=Enum: auto
  s16AngleParkLast : Inport  Port=2  OutDataTypeStr=int16
  s16Id : Inport  Port=3  OutDataTypeStr=int16
  s16Iq : Inport  Port=4  OutDataTypeStr=int16
  bEnMotorDriverLast : Inport  Port=5  OutDataTypeStr=boolean
  u32SpdRamp : Inport  Port=6  OutDataTypeStr=uint32
  Bus Creator : BusCreator  Inputs=4
  PiCtrl_Calc_D : Subsystem
  "PiCtrl_Calc_Q " : Subsystem
  parkangle_cal : Subsystem
  foc_state : Outport
  wires:
  eDirRun/1 -> parkangle_cal/1(eDirRun)
  u32SpdRamp/1 -> parkangle_cal/2(u32SpdRamp)
  PiCtrl_Calc_D/1(s16Vd) -> Bus Creator/2  "s16_foc_v_d"
  s16AngleParkLast/1 -> parkangle_cal/3(s16AngleParkLast)
  s16Id/1 -> PiCtrl_Calc_D/1(s16Id)
  parkangle_cal/1(s16AnglePark) -> Bus Creator/1  "s16_foc_parkangle"
  s16Iq/1 -> "PiCtrl_Calc_Q "/1(s16Iq)
  "PiCtrl_Calc_Q "/1(s16Vq) -> Bus Creator/3  "s16_foc_v_q"
  bEnMotorDriverLast/1 -> Bus Creator/4  "bEnMotorDriver"
  Bus Creator/1 -> foc_state/1

== system Foc_2024b/FieldOrientedControl/CurrentControl/MOTOR_STATE_RAMP_INIT ==
  s16AngleParkLast : Inport  OutDataTypeStr=int16
  s16Id : Inport  Port=2  OutDataTypeStr=int16
  s16Iq : Inport  Port=3  OutDataTypeStr=int16
  bEnMotorDriverLast : Inport  Port=4  OutDataTypeStr=boolean
  Compare To Constant : simulink/Logic and Bit Operations/Compare To Constant  relop===  const=false  OutDataTypeStr=boolean
  EnableDriver : Subsystem
  SetPiController : Subsystem
  Switch : Switch  Criteria=u2 ~= 0  SaturateOnIntegerOverflow=off  InputSameDT=off
  foc_state : Outport
  wires:
  bEnMotorDriverLast/1 -> [bEnMotorDriverLast]
  s16AngleParkLast/1 -> EnableDriver/1(s16AngleParkLast)
  [bEnMotorDriverLast] -> Compare To Constant/1
  s16Id/1 -> SetPiController/1(s16Id)
  [bEnMotorDriverLast] -> SetPiController/3(bEnMotorDriverLast)
  s16Iq/1 -> SetPiController/2(s16Iq)
  EnableDriver/1(foc_state) -> Switch/1
  Compare To Constant/1 -> Switch/2
  SetPiController/1(foc_state) -> Switch/3
  Switch/1 -> foc_state/1

== system Foc_2024b/FieldOrientedControl/CurrentControl/default ==
  bEnMotorDriverLast : Inport  OutDataTypeStr=boolean
  Bus Creator : BusCreator  Inputs=4
  Constant : Constant  Value=0  OutDataTypeStr=fixdt(1,16,15)
  Constant1 : Constant  Value=0  OutDataTypeStr=fixdt(1,16,15)
  Constant2 : Constant  Value=0  OutDataTypeStr=fixdt(1,16,15)
  foc_state : Outport
  wires:
  Constant/1 -> Bus Creator/1  "s16AnglePark"
  Constant1/1 -> Bus Creator/2  "s16Vd"
  Constant2/1 -> Bus Creator/3  "s16Vq"
  bEnMotorDriverLast/1 -> Bus Creator/4  "bEnMotorDriver"
  Bus Creator/1 -> foc_state/1

== system Foc_2024b/FieldOrientedControl/CurrentOffsets/OffsetDefault ==
  Action Port : ActionPort  ActionPortLabel=else
  Constant1 : Constant  Value=0  OutDataTypeStr=int32
  Constant2 : Constant  Value=0  OutDataTypeStr=int16
  Constant3 : Constant  Value=0  OutDataTypeStr=int16
  Constant4 : Constant  Value=0  OutDataTypeStr=int32
  s16PhaCurU : Outport  OutDataTypeStr=int16
  s16PhaCurV : Outport  Port=2  OutDataTypeStr=int16
  s32CurOffsetU : Outport  Port=3  OutDataTypeStr=int32
  s32CurOffsetV : Outport  Port=4  OutDataTypeStr=int32
  wires:
  Constant3/1 -> s16PhaCurV/1
  Constant4/1 -> s32CurOffsetV/1
  Constant1/1 -> s32CurOffsetU/1
  Constant2/1 -> s16PhaCurU/1
